simulink model "untitled"  (R2025a)
settings: Solver=VariableStepAuto  StartTime=0.0  StopTime=3  RelTol=1e-3
libraries: spsDCVoltageSourceLib x2, spsGroundLib x2, spsDCMachineLib x1, spsMultimeterLib x1, spsSeriesRLCBranchLib x1, sps_lib x1
settings Model: Creator=user  LastModifiedBy=user

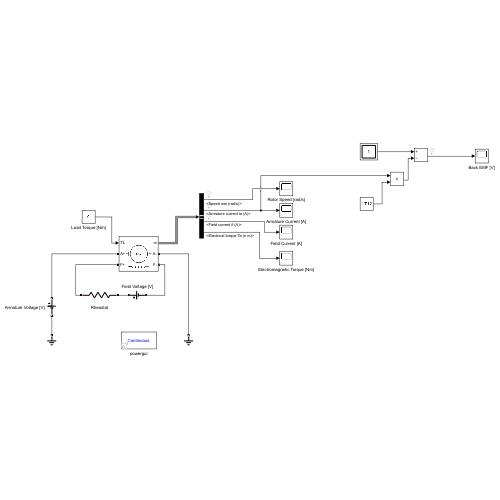
[thumbnail: Simulink's stored preview of the top-level diagram]
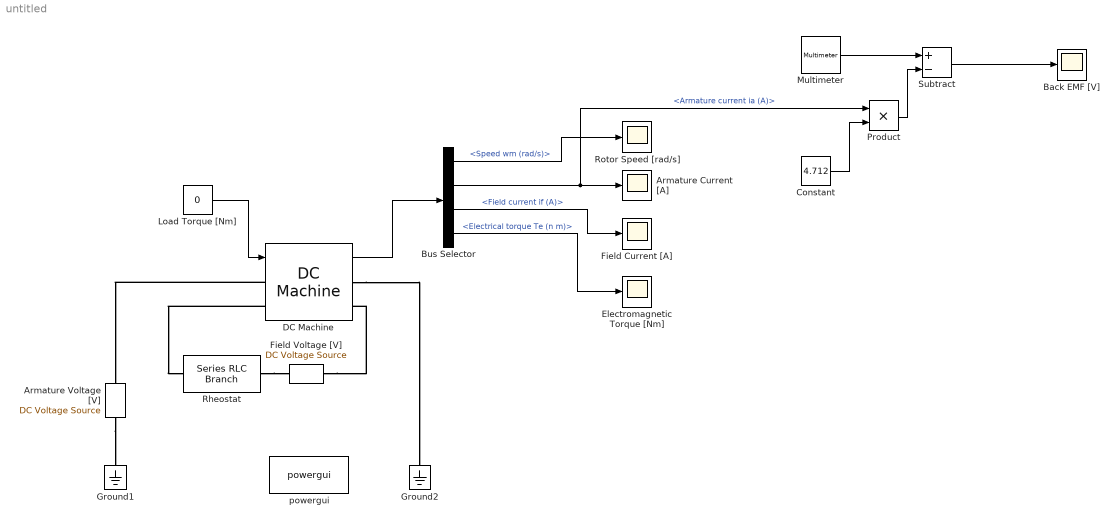
== system untitled ==
  Armature Current [A] : Scope
  Armature Voltage [V] : spsDCVoltageSourceLib/DC Voltage Source  Amplitude=500  Measurements=Voltage
  Back EMF [V] : Scope
      settings: DataLoggingVariableName=ScopeData4
  Bus Selector : BusSelector  OutputSignals=Speed wm (rad/s),Armature current ia (A),Field current if (A),Electrical torque Te (n m)
  Constant : Constant  Value=4.712
  DC Machine : spsDCMachineLib/DC Machine  PresetModel=05: 10HP 500V 1750RPM Field:300V  MechanicalLoad=Torque TL  FieldType=Wound  ShowDetailedParameters=on  MeasurementBus=off  RLa=[4.712 0.05277]  RLf=[180 71.47]  Laf=1.345  MachineConstant=Torque constant (N.m/A)  Ke=1.8  Kt=1.8  J=0.04251  Bm=0.003406  Tf=1.046  w0=1  Ifinit=1.30434782608696  TsPowergui=0  TsBlock=-1
  Electromagnetic Torque [Nm] : Scope
      settings: DataLoggingVariableName=ScopeData3
  Field Current [A] : Scope
      settings: DataLoggingVariableName=ScopeData2
  Field Voltage [V] : spsDCVoltageSourceLib/DC Voltage Source  Amplitude=300  Measurements=None
  Ground1 : spsGroundLib/Ground  LConnTagsString=a
  Ground2 : spsGroundLib/Ground  LConnTagsString=a
  Load Torque [Nm] : Constant  Value=0
  Multimeter : spsMultimeterLib/Multimeter  L=1  sel=1  yselected={}  Gain=1  OutputType=Complex  PlotAtSimulationStop=off  PhasorSimulation=off
  Product : Product
  Rheostat : spsSeriesRLCBranchLib/Series RLC Branch  LConnTagsString=__new0  RConnTagsString=__new0  BranchType=R  Resistance=50  Inductance=1e-3  SetiL0=off  InitialCurrent=0  Capacitance=1e-6  Setx0=off  InitialVoltage=0  Measurements=None
  Rotor Speed [rad/s] : Scope
  Subtract : Sum  Inputs=+-
  powergui : sps_lib/powergui  Priority=1  SimulationMode=Continuous  SampleTime=50e-6  frequency=60  Iterations=50  frequencyindice=0  Pbase=100e6  ErrMax=1e-4  UnitsV=kV  UnitsW=MW  buscounter=0  FunctionMessages=off  echomessages=off  EnableUseOfTLC=off  CurrentSourceSwitches=off  DisableSnubberDevices=off  DisableRonSwitches=off  DisableVfSwitches=off  DisplayEquations=off  AutomaticDiscreteSolvers=off  SolverType=Tustin/Backward Euler (TBE)  Interpol=off  ExternalGateDelay=off  methode=off  Ts=100  x0status=blocks  SPID=on  SwTol=0  HookPort=off  NonlinearTolerance=1e-4  nMaxIteration=100  ContinueOnMaxIteration=off  RestoreLinks=warning  ResistiveCurrentMeasurement=off  Frange=[0:2:500]  Ylog=off  Xlog=on  ShowGrid=off  save=off  variable=ZData  structure=0  ZoomFFT=off  StartTime=0.0  cycles=1  DisplayStyle=1  fundamental=60  FreqAxis=off  MaxFrequency=1000  frequencyindicesteady=1  RmsSteady=1  display=off
  wires:
  DC Machine/1 -> Bus Selector/1
  Bus Selector/1 -> Rotor Speed [rad/s]/1  "<Speed wm (rad/s)>"
  Bus Selector/2 -> Product/1, Armature Current [A]/1  "<Armature current ia (A)>"
  Bus Selector/4 -> Electromagnetic Torque [Nm]/1  "<Electrical torque Te (n m)>"
  Bus Selector/3 -> Field Current [A]/1  "<Field current if (A)>"
  Load Torque [Nm]/1 -> DC Machine/1
  Subtract/1 -> Back EMF [V]/1
  Multimeter/1 -> Subtract/1
  Product/1 -> Subtract/2
  Constant/1 -> Product/2
  connections:
  Armature Voltage [V]/LConn1 -- Ground1/LConn1
  DC Machine/LConn1 -- Armature Voltage [V]/RConn1
  Field Voltage [V]/LConn1 -- DC Machine/RConn2
  Rheostat/RConn1 -- Field Voltage [V]/RConn1
  DC Machine/LConn2 -- Rheostat/LConn1
  DC Machine/RConn1 -- Ground2/LConn1
